simulink model "PWM_simulink_sfunction"  (Simulink 7.6)
settings: Solver=ode23tb  StartTime=0.0  StopTime=5  MaxStep=0.00001  RelTol=1e-3
settings Model: Creator=user  LastModifiedBy=user

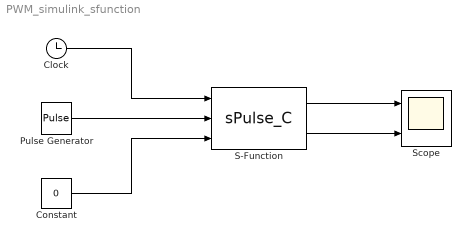
== system PWM_simulink_sfunction ==
  Clock : Clock
      settings: Decimation=10
  Constant : Constant  Value=0
  Pulse Generator : DiscretePulseGenerator  PulseType=Time based  Period=1/7200  PulseWidth=(0.35/360/60)*7200*100  PhaseDelay=0/360/60
  S-Function : S-Function  RequirementInfo="{}  %GIDa_7e879155_9ca7_43d6_bb3e_1e3ad60b9c5b"  FunctionName=sPulse_C  EnableBusSupport=off
  Scope : Scope  NumInputPorts=2
      settings: TimeRange=5  YMin=0~0  YMax=1~1
  wires:
  Constant/1 -> S-Function/3
  Clock/1 -> S-Function/1
  Pulse Generator/1 -> S-Function/2
  S-Function/1 -> Scope/1
  S-Function/2 -> Scope/2
